simulink model "verify_RadiationInclinedSurface_mdl"  (Simulink 8.2)
settings: Solver=FixedStepDiscrete  StartTime=31190400  StopTime=31276800  FixedStep=3600  RelTol=1e-3
libraries: carnot x4
settings Model: Creator=drhf  LastModifiedBy=drhf

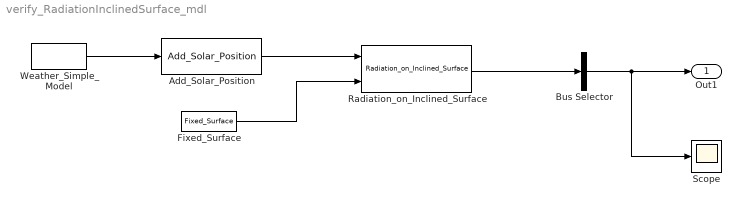
== system verify_RadiationInclinedSurface_mdl ==
  Add_Solar_Position : carnot/Weather/Add_Solar_Position  longi=0  lati=45  timezone=0
  Bus Selector : BusSelector  OutputSignals=Incidence_Angle_sun,Incidence_Angle_longitudinal,Incidence_Angle_transversal  OutputAsBus=on
  Fixed_Surface : carnot/Weather/Fixed_Surface  colangle=30  colazi=20  colrot=0
  Radiation_on_Inclined_Surface : carnot/Weather/Radiation_on_Inclined_Surface  sky=Perez 1990  reflect=0.2
  Scope : Scope
  Weather_Simple_Model : carnot/Weather/Weather_Simple_Model  lat=45  Ibn=900  Idg=100  tamb=5  deltaTsky=-6  rh=50  precip="10e-3/24/3600           % 10 mm in 24 h"  cloud=0.125  p=1013e2  vw=1  wdir=270
  Out1 : Outport
  wires:
  Weather_Simple_Model/1 -> Add_Solar_Position/1
  Bus Selector/1 -> Out1/1, Scope/1
  Fixed_Surface/1 -> Radiation_on_Inclined_Surface/2
  Add_Solar_Position/1 -> Radiation_on_Inclined_Surface/1
  Radiation_on_Inclined_Surface/1 -> Bus Selector/1
